simulink subsystem "Sensors"  (R2024b)
settings: Solver=VariableStepAuto  StartTime=0.0  StopTime=10.0  RelTol=1e-3
values from neighbouring files (symbols this model uses):
  OR_cg = [-2.50212 -2.5027 -2.50328 -2.50413 -2.50497 -2.50551 -2.50605 -2.50659 -2.5076 -2.5086 -2.50952 -2.51044 ... (1300 elements, 1300x1)]    [barrowaman.mat]
  sim_time = [0.01 0.02 0.03 0.04 0.05 0.06 0.07 0.08 0.09 0.1 0.11 0.12 ... (1300 elements, 1300x1)]    [barrowaman.mat]
undefined symbols (not defined in the file or in its folder): location, Ls1, samplingrate, Ss1, WMM2020
libraries: simulink x3, aerolibatmos2 x1, aerolibnav x1, aerolibgravity2 x1
settings Model: Creator=finnb  LastModifiedBy=finnb

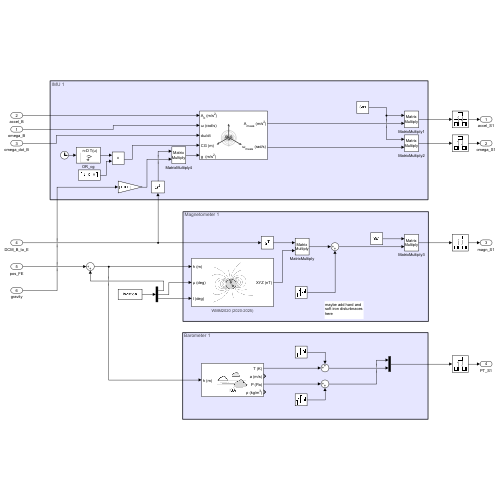
[thumbnail: Simulink's stored preview of the top-level diagram]
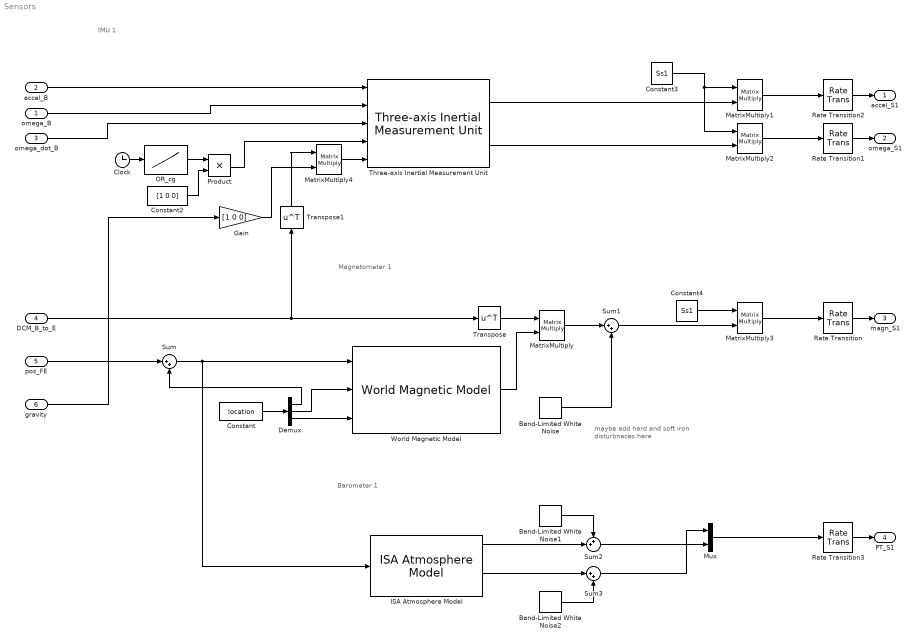
== system Sensors ==
  note: Barometer 1
  note: Magnetometer 1
  note: IMU 1
  note: maybe add hard and soft iron disturbnaces here
  omega_B : Inport
  accel_B : Inport  Port=2
  omega_dot_B : Inport  Port=3
  DCM_B_to_E : Inport  Port=4
  pos_FE : Inport  Port=5
  gravity : Inport  Port=6
  Band-Limited White Noise : simulink/Sources/Band-Limited White Noise  Cov=[0.001]  Ts=samplingrate  seed=[23341]
  Band-Limited White Noise1 : simulink/Sources/Band-Limited White Noise  Cov=[0.001]  Ts=samplingrate  seed=[2569]
  Band-Limited White Noise2 : simulink/Sources/Band-Limited White Noise  Cov=[0.001]  Ts=samplingrate  seed=[5781]
  Clock : Clock
  Constant : Constant  Value=location
  Constant2 : Constant  Value=[1 0 0]
  Constant3 : Constant  Value=Ss1
  Constant4 : Constant  Value=Ss1
  Demux : Demux  Outputs=3
  Gain : Gain  Gain=[1 0 0]
  ISA Atmosphere Model : aerolibatmos2/ISA Atmosphere Model  useExtended=on  action=Warning  custom=off  viscosityOut=off  g=9.80665  gamma=1.4  R=287.0531  L=0.0065  h_trop=11000  h_strat=20000  rho0=1.225  P0=101325  T0=288.15  h0=0  S=110.4  Tref=273.15  muref=1.716e-5
  MatrixMultiply{,1..4} (5 alike) : Product  Multiplication=Matrix(*)
  Mux : Mux  Inputs=2
  OR_cg : Lookup_n-D  NumberOfTableDimensions=1  BreakpointsForDimension1=sim_time  Table=OR_cg  InternalRulePriority=Speed  RndMeth=Simplest
  Product : Product
  Rate Transition{,1..3} (4 alike) : RateTransition  OutPortSampleTime=samplingrate
  Sum : Sum  Inputs=|++
  Sum1 : Sum  Inputs=|++
  Sum2 : Sum  Inputs=++|
  Sum3 : Sum  Inputs=|++
  Three-axis Inertial Measurement Unit : aerolibnav/Three-axis Inertial Measurement Unit  units=Metric (MKS)  imu=Ls1'  i_Ts=samplingrate  dtype_a=off  w_a=190  z_a=0.707  a_sf_cc=[1 0 0; 0 1 0; 0 0 1]  a_bias=[0 0 0]  a_sat="[-inf  -inf  -inf  inf inf inf]"  dtype_g=off  w_g=190  z_g=0.707  g_sf_cc=[1 0 0; 0 1 0; 0 0 1]  g_bias=[0 0 0]  g_sens=[0 0 0]  g_sat="[-inf  -inf  -inf  inf inf inf]"  i_rand=on  i_seeds=[23093 23094 23095 23096 23097 23098]  i_pow=[0.001 0.001 0.001 0.0001 0.0001 0.0001]
  Transpose : Math  Operator=transpose
  Transpose1 : Math  Operator=transpose
  World Magnetic Model : aerolibgravity2/World Magnetic Model  model=WMM2020 (2020-2025)  customFile='WMM2020.COF'  units=Metric (MKS)  time_in=off  month=January  day=1  year=2025  action=Error  h_out=off  dec_out=off  inc_out=off  ti_out=off
  accel_S1 : Outport
  omega_S1 : Outport  Port=2
  magn_S1 : Outport  Port=3
  PT_S1 : Outport  Port=4
  wires:
  accel_B/1 -> Three-axis Inertial Measurement Unit/1
  omega_B/1 -> Three-axis Inertial Measurement Unit/2
  omega_dot_B/1 -> Three-axis Inertial Measurement Unit/3
  OR_cg/1 -> Product/1
  MatrixMultiply4/1 -> Three-axis Inertial Measurement Unit/5
  Three-axis Inertial Measurement Unit/1 -> MatrixMultiply1/2
  Three-axis Inertial Measurement Unit/2 -> MatrixMultiply2/2
  Clock/1 -> OR_cg/1
  Product/1 -> Three-axis Inertial Measurement Unit/4
  Constant2/1 -> Product/2
  Constant/1 -> Demux/1
  Demux/3 -> World Magnetic Model/3
  Demux/2 -> World Magnetic Model/2
  Sum/1 -> World Magnetic Model/1, ISA Atmosphere Model/1
  Demux/1 -> Sum/2
  pos_FE/1 -> Sum/1
  DCM_B_to_E/1 -> Transpose1/1, Transpose/1
  Transpose/1 -> MatrixMultiply/1
  World Magnetic Model/1 -> MatrixMultiply/2
  MatrixMultiply/1 -> Sum1/1
  Band-Limited White Noise/1 -> Sum1/2
  Rate Transition/1 -> magn_S1/1
  Sum1/1 -> MatrixMultiply3/2
  Rate Transition1/1 -> omega_S1/1
  Rate Transition2/1 -> accel_S1/1
  MatrixMultiply1/1 -> Rate Transition2/1
  Constant3/1 -> MatrixMultiply2/1, MatrixMultiply1/1
  MatrixMultiply2/1 -> Rate Transition1/1
  MatrixMultiply3/1 -> Rate Transition/1
  Mux/1 -> Rate Transition3/1
  ISA Atmosphere Model/1 -> Sum2/2
  ISA Atmosphere Model/3 -> Sum3/1
  Band-Limited White Noise1/1 -> Sum2/1
  Sum2/1 -> Mux/2
  Sum3/1 -> Mux/1
  Band-Limited White Noise2/1 -> Sum3/2
  Constant4/1 -> MatrixMultiply3/1
  Rate Transition3/1 -> PT_S1/1
  Gain/1 -> MatrixMultiply4/2
  gravity/1 -> Gain/1
  Transpose1/1 -> MatrixMultiply4/1
